simulink model "PassengerCar"  (R2019b)
settings: Solver=ode1  StartTime=0  StopTime=25  FixedStep=1.0000000000000000e-003  RelTol=1e-3
InitFcn:
  | sampleTime = str2double(get_param(bdroot, 'FixedStep'));
undefined symbols (not defined in the file or in its folder): AccPedalPos, BrakePedalPos, BrakeSwitch, DiscIntNeverNeededParam, DYNA4, EngSpd, IgnitionSwitch, InitialGear, InitialSpeed, IntendedEngTrq, LeftIndicator, MainBrakePress, MaxGear, MDL, MinGear, RefAcc, RefLane, RefLatPos, RefPath, RefPathCurv, RefSpd, RefSpdPreview, RefSpdRetrospect, RightIndicator, SteeringWheelAng, SteeringWheelTrq, UserDefinedRefValue, vm_const
libraries: UtilitiesLibrary x31, simulink x18, WheelSystemModules x13, LongitudinalControllerModules x13, LateralControllerModules x7, AnimationBusselectorModules x5, EnvironmentModules x5, BasicEngineControlModules x5, MiscellaneousControlModules x5, Animation3Modules x4, AuxiliariesModules x4, TireModules x4
(part 9 of 39)

== system PassengerCar/Vehicle/BrakeSystem/BrakeSystemPhysics ==
  fromBrakeControlCoordinator : Inport
  fromCTRL : Inport  Port=2
  fromBrakeSystemControlUnit : Inport  Port=3
  BrakeSystemPhysicsOutput : Subsystem  Tag=TESIS DYNAware Interface Block  mask{NeedsUpdate=off, SignalInfo=|}
      mask SignalInfo=|
      | {
      |   "Version": "4.6",
      |   "MuxedOutputBusName": "BrakeSystemPhysics",
      |   "MuxedInputBusName": "input",
      |   "MuxedInputSelected": false,
      |   "MuxedOutputSelected": true,
      |   "SignalData": [
      |     {
      |       "initialValue": "0.0",
      |       "name": "WheelBrakePressActive[0;1]",
      |       "comment": "",
      |       "minString": "",
      |       "maxString": "",
      |       "width": 1,
      |       "dataType": 0,
      |       "signalType": 0,
      |       "createSignal": false,
      |       "outputName": "WheelBrakePressActive[0;1]",
      |       "generateSignalAccessBlock": false,
      |       "accessId": "$(parentId).$(blockName).$(outputName)"
      |     },
      |     {
      |       "initialValue": "0.0",
      |       "name": "MaxMainBrakePress[Pa]",
      |       "comment": "",
      |       "minString": "",
      |       "maxString": "",
      |       "width": 1,
      |       "dataType": 0,
      |       "signalType": 0,
      |       "createSignal": false,
      |       "outputName": "MaxMainBrakePress[Pa]",
      |       "generateSignalAccessBlock": false,
      |       "accessId": "$(parentId).$(blockName).$(outputName)"
      |     },
      |     {
      |       "initialValue": "0.0",
      |       "name": "MainBrakePress[Pa]",
      |       "comment": "",
      |       "minString": "",
      |       "maxString": "",
      |       "width": 1,
      |       "dataType": 0,
      |       "signalType": 0,
      |       "createSignal": false,
      |       "outputName": "MainBrakePress[Pa]",
      |       "generateSignalAccessBlock": false,
      |       "accessId": "$(parentId).$(blockName).$(outputName)"
      |     },
      |     {
      |       "initialValue": "",
      |       "name": "FrontLeftWheelBrakePress[Pa]",
      |       "comment": "",
      |       "minString": "",
      |       "maxString": "",
      |       "width": 1,
      |       "dataType": 0,
      |       "signalType": 0,
      |       "createSignal": false,
      |       "outputName": "FrontLeftWheelBrakePress[Pa]",
      |       "generateSignalAccessBlock": false,
      |       "accessId": "$(parentId).$(blockName).$(outputName)"
      |     },
      |     {
      |       "initialValue": "",
      |       "name": "FrontRightWheelBrakePress[Pa]",
      |       "comment": "",
      |       "minString": "",
      |       "maxString": "",
      |       "width": 1,
      |       "dataType": 0,
      |       "signalType": 0,
      |       "createSignal": false,
      |       "outputName": "FrontRightWheelBrakePress[Pa]",
      |       "generateSignalAccessBlock": false,
      |       "accessId": "$(parentId).$(blockName).$(outputName)"
      |     },
      |     {
      |       "initialValue": "",
      |       "name": "RearLeftWheelBrakePress[Pa]",
      |       "comment": "",
      |       "minString": "",
      |       "maxString": "",
      |       "width": 1,
      |       "dataType": 0,
      |       "signalType": 0,
      |       "createSignal": false,
      |       "outputName": "RearLeftWheelBrakePress[Pa]",
      |       "generateSignalAccessBlock": false,
      |       "accessId": "$(parentId).$(blockName).$(outputName)"
      |     },
      |     {
      |       "initialValue": "",
      |       "name": "RearRightWheelBrakePress[Pa]",
      |       "comment": "",
      |       "minString": "",
      |       "maxString": "",
      |       "width": 1,
      |       "dataType": 0,
      |       "signalType": 0,
      |       "createSignal": false,
      |       "outputName": "RearRightWheelBrakePress[Pa]",
      |       "generateSignalAccessBlock": false,
      |       "accessId": "$(parentId).$(blockName).$(outputName)"
      |     },
      |     {
      |       "initialValue": "",
      |       "name": "Rear2LeftWheelBrakePress[Pa]",
      |       "comment": "",
      |       "minString": "",
      |       "maxString": "",
      |       "width": 1,
      |       "dataType": 0,
      |       "signalType": 0,
      |       "createSignal": false,
      |       "outputName": "Rear2LeftWheelBrakePress[Pa]",
      |       "generateSignalAccessBlock": false,
      |       "accessId": "$(parentId).$(blockName).$(outputName)"
      |     },
      |     {
      |       "initialValue": "",
      |       "name": "Rear2RightWheelBrakePress[Pa]",
      |       "comment": "",
      |       "minString": "",
      |       "maxString": "",
      |       "width": 1,
      |       "dataType": 0,
      |       "signalType": 0,
      |       "createSignal": false,
      |       "outputName": "Rear2RightWheelBrakePress[Pa]",
      |       "generateSignalAccessBlock": false,
      |       "accessId": "$(parentId).$(blockName).$(outputName)"
      |     },
      |     {
      |       "initialValue": "",
      |       "name": "Rear3LeftWheelBrakePress[Pa]",
      |       "comment": "",
      |       "minString": "",
      |       "maxString": "",
      |       "width": 1,
      |       "dataType": 0,
      |       "signalType": 0,
      |       "createSignal": false,
      |       "outputName": "Rear3LeftWheelBrakePress[Pa]",
      |       "generateSignalAccessBlock": false,
      |       "accessId": "$(parentId).$(blockName).$(outputName)"
      |     },
      |     {
      |       "initialValue": "",
      |       "name": "Rear3RightWheelBrakePress[Pa]",
      |       "comment": "",
      |       "minString": "",
      |       "maxString": "",
      |       "width": 1,
      |       "dataType": 0,
      |       "signalType": 0,
      |       "createSignal": false,
      |       "outputName": "Rear3RightWheelBrakePress[Pa]",
      |       "generateSignalAccessBlock": false,
      |       "accessId": "$(parentId).$(blockName).$(outputName)"
      |     }
      |   ]
      | }
      mask prompts: NeedsUpdate "Specify, if subsystem content needs to be updated"; SignalInfo "Signal Info (json)"
      mask help: DYNA4 Interface Block Version 4.6
      mask init:
      | blockName = get_param(gcbh, 'Name');
      | parentId = DYNA4.ModelHandling.AccessID.getFromHierarchy(gcbh);
      | TD.InterfaceBlock.ModelCallbacks.GenerateContent(gcb);
      settings: DeleteFcn=TD.InterfaceBlock.ModelCallbacks.CloseGUI( gcbh );  NameChangeFcn=TD.InterfaceBlock.ModelCallbacks.BlockRenamedHandler(gcbh);  OpenFcn=TD.InterfaceBlock.ModelCallbacks.OpenGUI( gcbh );  CloseFcn=TD.InterfaceBlock.ModelCallbacks.CloseGUI( gcbh );
      mask Display:
      | image('InterfaceBlock.png','center');
      | port_label('input',1, 'WheelBrakePressActive[0;1]');
      | port_label('input',2, 'MaxMainBrakePress[Pa]');
      | port_label('input',3, 'MainBrakePress[Pa]');
      | port_label('input',4, 'FrontLeftWheelBrakePress[Pa]');
      | port_label('input',5, 'FrontRightWheelBrakePress[Pa]');
      | port_label('input',6, 'RearLeftWheelBrakePress[Pa]');
      | port_label('input',7, 'RearRightWheelBrakePress[Pa]');
      | port_label('input',8, 'Rear2LeftWheelBrakePress[Pa]');
      | port_label('input',9, 'Rear2RightWheelBrakePress[Pa]');
      | port_label('input',10, 'Rear3LeftWheelBrakePress[Pa]');
      | port_label('input',11, 'Rear3RightWheelBrakePress[Pa]');
      | port_label('output',1, 'BrakeSystemPhysics');
  Compare To Constant : simulink/Logic and Bit Operations/Compare To Constant  relop=~=  const=double(DYNA4.Vehicle.BrakeSystem.BrakeSwitch.WHEEL_BRAKE_PRESSURES)  OutDataTypeStr=boolean
  Data Type Conversion : DataTypeConversion  OutDataTypeStr=double
  Demux : Demux  Outputs=8
  DynaComponentInfo : Subsystem  Tag=DynaComponentInfo
      mask init:
      | data= get_param(gcb, 'UserData');
      settings: OpenFcn=DYNA4.ModelHandling.Component.ShowEditComponentInformationDialog(gcb);
      mask Display: disp(['Type = ', data.type, '\nGroup = ', data.group, '\nName = ', data.name ])
  InputFromBrakeControlCoordinator : Subsystem  Tag=TESIS DYNAware Interface Block  mask{NeedsUpdate=off, SignalInfo=|}
      mask SignalInfo=|
      | {
      |   "Version": "4.6",
      |   "MuxedOutputBusName": "output",
      |   "MuxedInputBusName": "fromBrakeControlCoordinator",
      |   "MuxedInputSelected": true,
      |   "MuxedOutputSelected": false,
      |   "SignalData": [
      |     {
      |       "initialValue": "",
      |       "name": "BrakeSwitch[1;3]",
      |       "comment": "",
      |       "minString": "",
      |       "maxString": "",
      |       "width": -1,
      |       "dataType": 0,
      |       "signalType": 0,
      |       "createSignal": false,
      |       "outputName": "BrakeSwitch[1;3]",
      |       "generateSignalAccessBlock": false,
      |       "accessId": "$(parentId).$(blockName).$(outputName)"
      |     },
      |     {
      |       "initialValue": "",
      |       "name": "MainBrakePress[Pa]",
      |       "comment": "",
      |       "minString": "",
      |       "maxString": "",
      |       "width": -1,
      |       "dataType": 0,
      |       "signalType": 0,
      |       "createSignal": false,
      |       "outputName": "MainBrakePress[Pa]",
      |       "generateSignalAccessBlock": false,
      |       "accessId": "$(parentId).$(blockName).$(outputName)"
      |     }
      |   ]
      | }
      mask prompts: NeedsUpdate "Specify, if subsystem content needs to be updated"; SignalInfo "Signal Info (json)"
      mask help: DYNA4 Interface Block Version 4.6
      mask init:
      | blockName = get_param(gcbh, 'Name');
      | parentId = DYNA4.ModelHandling.AccessID.getFromHierarchy(gcbh);
      | TD.InterfaceBlock.ModelCallbacks.GenerateContent(gcb);
      settings: DeleteFcn=TD.InterfaceBlock.ModelCallbacks.CloseGUI( gcbh );  NameChangeFcn=TD.InterfaceBlock.ModelCallbacks.BlockRenamedHandler(gcbh);  OpenFcn=TD.InterfaceBlock.ModelCallbacks.OpenGUI( gcbh );  CloseFcn=TD.InterfaceBlock.ModelCallbacks.CloseGUI( gcbh );
      mask Display:
      | image('InterfaceBlock.png','center');
      | port_label('input',1, 'fromBrakeControlCoordinator');
      | port_label('output',1, 'BrakeSwitch[1;3]');
      | port_label('output',2, 'MainBrakePress[Pa]');
  InputFromCTRL : Subsystem  Tag=TESIS DYNAware Interface Block  mask{NeedsUpdate=off, SignalInfo=|}
      mask SignalInfo=|
      | {
      |   "Version": "4.6",
      |   "MuxedOutputBusName": "output",
      |   "MuxedInputBusName": "fromCTRL",
      |   "MuxedInputSelected": true,
      |   "MuxedOutputSelected": false,
      |   "SignalData": {
      |     "initialValue": "0.0",
      |     "name": "CTRL.LongitudinalControl.BrakePedalPos[0_1]",
      |     "comment": "",
      |     "minString": "",
      |     "maxString": "",
      |     "width": 1,
      |     "dataType": 0,
      |     "signalType": 0,
      |     "createSignal": false,
      |     "outputName": "BrakePedalPos[0_1]",
      |     "generateSignalAccessBlock": false,
      |     "accessId": "$(parentId).$(blockName).$(outputName)"
      |   }
      | }
      mask prompts: NeedsUpdate "Specify, if subsystem content needs to be updated"; SignalInfo "Signal Info (json)"
      mask help: DYNA4 Interface Block Version 4.6
      mask init:
      | blockName = get_param(gcbh, 'Name');
      | parentId = DYNA4.ModelHandling.AccessID.getFromHierarchy(gcbh);
      | TD.InterfaceBlock.ModelCallbacks.GenerateContent(gcb);
      settings: DeleteFcn=TD.InterfaceBlock.ModelCallbacks.CloseGUI( gcbh );  NameChangeFcn=TD.InterfaceBlock.ModelCallbacks.BlockRenamedHandler(gcbh);  OpenFcn=TD.InterfaceBlock.ModelCallbacks.OpenGUI( gcbh );  CloseFcn=TD.InterfaceBlock.ModelCallbacks.CloseGUI( gcbh );
      mask Display:
      | image('InterfaceBlock.png','center');
      | port_label('input',1, 'fromCTRL');
      | port_label('output',1, 'BrakePedalPos[0_1]');
  TabledBrakeHydraulics : BrakeSystemModules/TabledBrakeHydraulics  Tag=vedynaBrkHydMask  local_comp_inst=1  system_comp_inst=1  DATA_NODE=MDL.Vehicle.BrakeSystem.BrakeSystemPhysics.TabledBrakeHydraulics  sample_time=-1
  Terminator : Terminator
  BrakeSystemPhysics : Outport  VectorParamsAs1DForOutWhenUnconnected=off
  wires:
  Demux/1 -> BrakeSystemPhysicsOutput/4(FrontLeftWheelBrakePress[Pa]___UNIQUE_1)
  Demux/2 -> BrakeSystemPhysicsOutput/5(FrontRightWheelBrakePress[Pa]___UNIQUE_1)
  Demux/3 -> BrakeSystemPhysicsOutput/6(RearLeftWheelBrakePress[Pa]___UNIQUE_1)
  Demux/4 -> BrakeSystemPhysicsOutput/7(RearRightWheelBrakePress[Pa]___UNIQUE_1)
  Demux/5 -> BrakeSystemPhysicsOutput/8(Rear2LeftWheelBrakePress[Pa]___UNIQUE_1)
  Demux/6 -> BrakeSystemPhysicsOutput/9(Rear2RightWheelBrakePress[Pa]___UNIQUE_1)
  Demux/7 -> BrakeSystemPhysicsOutput/10(Rear3LeftWheelBrakePress[Pa]___UNIQUE_1)
  Demux/8 -> BrakeSystemPhysicsOutput/11(Rear3RightWheelBrakePress[Pa]___UNIQUE_1)
  InputFromCTRL/1(BrakePedalPos[0_1]___UNIQUE_1) -> TabledBrakeHydraulics/2
  fromCTRL/1 -> InputFromCTRL/1(fromCTRL)
  TabledBrakeHydraulics/3 -> Demux/1
  TabledBrakeHydraulics/2 -> BrakeSystemPhysicsOutput/3(MainBrakePress[Pa]___UNIQUE_1)
  TabledBrakeHydraulics/1 -> BrakeSystemPhysicsOutput/2(MaxMainBrakePress[Pa]___UNIQUE_1)
  BrakeSystemPhysicsOutput/1(BrakeSystemPhysics___UNIQUE_1) -> BrakeSystemPhysics/1
  fromBrakeControlCoordinator/1 -> InputFromBrakeControlCoordinator/1(fromBrakeControlCoordinator)
  InputFromBrakeControlCoordinator/1(BrakeSwitch[1;3]___UNIQUE_1) -> TabledBrakeHydraulics/1, Compare To Constant/1
  InputFromBrakeControlCoordinator/2(MainBrakePress[Pa]___UNIQUE_1) -> TabledBrakeHydraulics/3
  fromBrakeSystemControlUnit/1 -> Terminator/1
  Compare To Constant/1 -> Data Type Conversion/1
  Data Type Conversion/1 -> BrakeSystemPhysicsOutput/1(WheelBrakePressActive[0;1]___UNIQUE_1)

== system PassengerCar/Vehicle/BrakeSystem/BrakeSystemPhysicsOutput ==
  MaxMainBrakePress[Pa]___UNIQUE_1 : Inport  Description=|  PortDimensions=[1]
      | <name>MaxMainBrakePress[Pa]</name>
      | <comment></comment>
  MainBrakePress[Pa]___UNIQUE_1 : Inport  Description=|  Port=2  PortDimensions=[1]
      | <name>MainBrakePress[Pa]</name>
      | <comment></comment>
  FrontLeftWheelBrakePress[Pa]___UNIQUE_1 : Inport  Description=|  Port=3
      | <name>FrontLeftWheelBrakePress[Pa]</name>
      | <comment></comment>
  FrontRightWheelBrakePress[Pa]___UNIQUE_1 : Inport  Description=|  Port=4
      | <name>FrontRightWheelBrakePress[Pa]</name>
      | <comment></comment>
  RearLeftWheelBrakePress[Pa]___UNIQUE_1 : Inport  Description=|  Port=5
      | <name>RearLeftWheelBrakePress[Pa]</name>
      | <comment></comment>
  RearRightWheelBrakePress[Pa]___UNIQUE_1 : Inport  Description=|  Port=6
      | <name>RearRightWheelBrakePress[Pa]</name>
      | <comment></comment>
  Rear2LeftWheelBrakePress[Pa]___UNIQUE_1 : Inport  Description=|  Port=7
      | <name>Rear2LeftWheelBrakePress[Pa]</name>
      | <comment></comment>
  Rear2RightWheelBrakePress[Pa]___UNIQUE_1 : Inport  Description=|  Port=8
      | <name>Rear2RightWheelBrakePress[Pa]</name>
      | <comment></comment>
  Rear3LeftWheelBrakePress[Pa]___UNIQUE_1 : Inport  Description=|  Port=9
      | <name>Rear3LeftWheelBrakePress[Pa]</name>
      | <comment></comment>
  Rear3RightWheelBrakePress[Pa]___UNIQUE_1 : Inport  Description=|  Port=10
      | <name>Rear3RightWheelBrakePress[Pa]</name>
      | <comment></comment>
  WheelBrakePressSource[-]___UNIQUE_1 : Inport  Description=|  Port=11  PortDimensions=[1]
      | <name>WheelBrakePressSource[-]</name>
      | <comment></comment>
  __TDD__BrakeSystem.FrontLeftWheelBrakePress[Pa] : Demux  Outputs=1
  __TDD__BrakeSystem.FrontRightWheelBrakePress[Pa] : Demux  Outputs=1
  __TDD__BrakeSystem.MainBrakePress[Pa] : Demux  Outputs=[1]
  __TDD__BrakeSystem.MaxMainBrakePress[Pa] : Demux  Outputs=[1]
  __TDD__BrakeSystem.Rear2LeftWheelBrakePress[Pa] : Demux  Outputs=1
  __TDD__BrakeSystem.Rear2RightWheelBrakePress[Pa] : Demux  Outputs=1
  __TDD__BrakeSystem.Rear3LeftWheelBrakePress[Pa] : Demux  Outputs=1
  __TDD__BrakeSystem.Rear3RightWheelBrakePress[Pa] : Demux  Outputs=1
  __TDD__BrakeSystem.RearLeftWheelBrakePress[Pa] : Demux  Outputs=1
  __TDD__BrakeSystem.RearRightWheelBrakePress[Pa] : Demux  Outputs=1
  __TDD__BrakeSystem.WheelBrakePressSource[-] : Demux  Outputs=[1]
  __TDO__BrakeSystem : BusCreator  Inputs=11
  BrakeSystem___UNIQUE_1 : Outport  Description=|  VectorParamsAs1DForOutWhenUnconnected=off
      | <name>MaxMainBrakePress[Pa]</name>
      | <comment></comment>
  wires:
  MaxMainBrakePress[Pa]___UNIQUE_1/1 -> __TDD__BrakeSystem.MaxMainBrakePress[Pa]/1  "MaxMainBrakePress[Pa]"
  __TDD__BrakeSystem.MaxMainBrakePress[Pa]/1 -> __TDO__BrakeSystem/1  "MaxMainBrakePress[Pa]"
  MainBrakePress[Pa]___UNIQUE_1/1 -> __TDD__BrakeSystem.MainBrakePress[Pa]/1  "MainBrakePress[Pa]"
  __TDD__BrakeSystem.MainBrakePress[Pa]/1 -> __TDO__BrakeSystem/2  "MainBrakePress[Pa]"
  FrontLeftWheelBrakePress[Pa]___UNIQUE_1/1 -> __TDD__BrakeSystem.FrontLeftWheelBrakePress[Pa]/1  "FrontLeftWheelBrakePress[Pa]"
  __TDD__BrakeSystem.FrontLeftWheelBrakePress[Pa]/1 -> __TDO__BrakeSystem/3  "FrontLeftWheelBrakePress[Pa]"
  FrontRightWheelBrakePress[Pa]___UNIQUE_1/1 -> __TDD__BrakeSystem.FrontRightWheelBrakePress[Pa]/1  "FrontRightWheelBrakePress[Pa]"
  __TDD__BrakeSystem.FrontRightWheelBrakePress[Pa]/1 -> __TDO__BrakeSystem/4  "FrontRightWheelBrakePress[Pa]"
  RearLeftWheelBrakePress[Pa]___UNIQUE_1/1 -> __TDD__BrakeSystem.RearLeftWheelBrakePress[Pa]/1  "RearLeftWheelBrakePress[Pa]"
  __TDD__BrakeSystem.RearLeftWheelBrakePress[Pa]/1 -> __TDO__BrakeSystem/5  "RearLeftWheelBrakePress[Pa]"
  RearRightWheelBrakePress[Pa]___UNIQUE_1/1 -> __TDD__BrakeSystem.RearRightWheelBrakePress[Pa]/1  "RearRightWheelBrakePress[Pa]"
  __TDD__BrakeSystem.RearRightWheelBrakePress[Pa]/1 -> __TDO__BrakeSystem/6  "RearRightWheelBrakePress[Pa]"
  Rear2LeftWheelBrakePress[Pa]___UNIQUE_1/1 -> __TDD__BrakeSystem.Rear2LeftWheelBrakePress[Pa]/1  "Rear2LeftWheelBrakePress[Pa]"
  __TDD__BrakeSystem.Rear2LeftWheelBrakePress[Pa]/1 -> __TDO__BrakeSystem/7  "Rear2LeftWheelBrakePress[Pa]"
  Rear2RightWheelBrakePress[Pa]___UNIQUE_1/1 -> __TDD__BrakeSystem.Rear2RightWheelBrakePress[Pa]/1  "Rear2RightWheelBrakePress[Pa]"
  __TDD__BrakeSystem.Rear2RightWheelBrakePress[Pa]/1 -> __TDO__BrakeSystem/8  "Rear2RightWheelBrakePress[Pa]"
  Rear3LeftWheelBrakePress[Pa]___UNIQUE_1/1 -> __TDD__BrakeSystem.Rear3LeftWheelBrakePress[Pa]/1  "Rear3LeftWheelBrakePress[Pa]"
  __TDD__BrakeSystem.Rear3LeftWheelBrakePress[Pa]/1 -> __TDO__BrakeSystem/9  "Rear3LeftWheelBrakePress[Pa]"
  Rear3RightWheelBrakePress[Pa]___UNIQUE_1/1 -> __TDD__BrakeSystem.Rear3RightWheelBrakePress[Pa]/1  "Rear3RightWheelBrakePress[Pa]"
  __TDD__BrakeSystem.Rear3RightWheelBrakePress[Pa]/1 -> __TDO__BrakeSystem/10  "Rear3RightWheelBrakePress[Pa]"
  WheelBrakePressSource[-]___UNIQUE_1/1 -> __TDD__BrakeSystem.WheelBrakePressSource[-]/1
  __TDD__BrakeSystem.WheelBrakePressSource[-]/1 -> __TDO__BrakeSystem/11  "WheelBrakePressSource[-]"
  __TDO__BrakeSystem/1 -> BrakeSystem___UNIQUE_1/1  "BrakeSystem"

== system PassengerCar/Vehicle/BrakeSystem/DynaComponentInfo ==

== system PassengerCar/Vehicle/BrakeSystem/Signal Prioritizer ==
  BrakeControlCoordinator : Inport
  BrakeSystemControlUnit : Inport  Port=2
  BrakeSystemPhysics : Inport  Port=3
  Add : Sum
  Bus Creator : BusCreator  Inputs=8
  Bus Selector : BusSelector  OutputSignals=FrontLeftWheelBrakePress[Pa],FrontRightWheelBrakePress[Pa],RearLeftWheelBrakePress[Pa],RearRightWheelBrakePress[Pa],Rear2LeftWheelBrakePress[Pa],Rear2RightWheelBrakePress[Pa],Rear3LeftWheelBrakePress[Pa],Rear3RightWheelBrakePress[Pa],WheelBrakePressActive[0;1]
  Bus Selector1 : BusSelector  OutputSignals=FrontLeftWheelBrakePress[Pa],FrontRightWheelBrakePress[Pa],RearLeftWheelBrakePress[Pa],RearRightWheelBrakePress[Pa],Rear2LeftWheelBrakePress[Pa],Rear2RightWheelBrakePress[Pa],Rear3LeftWheelBrakePress[Pa],Rear3RightWheelBrakePress[Pa],WheelBrakePressActive[0;1]
  Bus Selector2 : BusSelector  OutputSignals=FrontLeftWheelBrakePress[Pa],FrontRightWheelBrakePress[Pa],RearLeftWheelBrakePress[Pa],RearRightWheelBrakePress[Pa],Rear2LeftWheelBrakePress[Pa],Rear2RightWheelBrakePress[Pa],Rear3LeftWheelBrakePress[Pa],Rear3RightWheelBrakePress[Pa],WheelBrakePressActive[0;1]
  Compare To Zero : simulink/Logic and Bit Operations/Compare To Zero  relop===  OutDataTypeStr=boolean
  Constant : Constant  Value=1:4
  Constant1 : Constant  Value=[1:3, -1]
  Constant2 : Constant
  Constant3 : Constant  Value=zeros(8,1)  VectorParams1D=off
  Demux : Demux  Outputs=8
  Gain : Gain  Gain=4
  MinMax : MinMax
  Product : Product  Tag=productActive
  Selector : Selector  NumberOfDimensions=2  InputPortWidth=3  IndexOptions=Select all,Starting index (port)  Indices=[1 3]  OutputSizes=1,1
  Selector1 : Selector  NumberOfDimensions=2  InputPortWidth=3  IndexOptions=Select all,Starting index (port)  Indices=[1 3]  OutputSizes=1,1
  Vector Concatenate : Concatenate  NumInputs=4
  Vector Concatenate1 : Concatenate  NumInputs=4  Mode=Multidimensional array  ConcatenateDimension=2
  Vector Concatenate2 : Concatenate  NumInputs=8
  Vector Concatenate3 : Concatenate  NumInputs=8
  Vector Concatenate4 : Concatenate  NumInputs=8
  ControlSignals : Outport  VectorParamsAs1DForOutWhenUnconnected=off
  SelectedInput : Outport  Port=2  VectorParamsAs1DForOutWhenUnconnected=off
  wires:
  Vector Concatenate4/1 -> Vector Concatenate1/3
  Bus Selector2/9 -> Vector Concatenate/3  "<WheelBrakePressActive[0;1]>"
  BrakeSystemPhysics/1 -> Bus Selector2/1
  Bus Selector2/8 -> Vector Concatenate4/8  "<Rear3RightWheelBrakePress[Pa]>"
  Bus Selector2/7 -> Vector Concatenate4/7  "<Rear3LeftWheelBrakePress[Pa]>"
  Bus Selector2/6 -> Vector Concatenate4/6  "<Rear2RightWheelBrakePress[Pa]>"
  Bus Selector2/5 -> Vector Concatenate4/5  "<Rear2LeftWheelBrakePress[Pa]>"
  Bus Selector2/4 -> Vector Concatenate4/4  "<RearRightWheelBrakePress[Pa]>"
  Bus Selector2/3 -> Vector Concatenate4/3  "<RearLeftWheelBrakePress[Pa]>"
  Bus Selector2/2 -> Vector Concatenate4/2  "<FrontRightWheelBrakePress[Pa]>"
  Bus Selector2/1 -> Vector Concatenate4/1  "<FrontLeftWheelBrakePress[Pa]>"
  Vector Concatenate3/1 -> Vector Concatenate1/2
  Bus Selector1/9 -> Vector Concatenate/2  "<WheelBrakePressActive[0;1]>"
  BrakeSystemControlUnit/1 -> Bus Selector1/1
  Bus Selector1/8 -> Vector Concatenate3/8  "<Rear3RightWheelBrakePress[Pa]>"
  Bus Selector1/7 -> Vector Concatenate3/7  "<Rear3LeftWheelBrakePress[Pa]>"
  Bus Selector1/6 -> Vector Concatenate3/6  "<Rear2RightWheelBrakePress[Pa]>"
  Bus Selector1/5 -> Vector Concatenate3/5  "<Rear2LeftWheelBrakePress[Pa]>"
  Bus Selector1/4 -> Vector Concatenate3/4  "<RearRightWheelBrakePress[Pa]>"
  Bus Selector1/3 -> Vector Concatenate3/3  "<RearLeftWheelBrakePress[Pa]>"
  Bus Selector1/2 -> Vector Concatenate3/2  "<FrontRightWheelBrakePress[Pa]>"
  Bus Selector1/1 -> Vector Concatenate3/1  "<FrontLeftWheelBrakePress[Pa]>"
  Vector Concatenate2/1 -> Vector Concatenate1/1
  Bus Selector/9 -> Vector Concatenate/1  "<WheelBrakePressActive[0;1]>"
  BrakeControlCoordinator/1 -> Bus Selector/1
  Bus Selector/8 -> Vector Concatenate2/8  "<Rear3RightWheelBrakePress[Pa]>"
  Bus Selector/7 -> Vector Concatenate2/7  "<Rear3LeftWheelBrakePress[Pa]>"
  Bus Selector/6 -> Vector Concatenate2/6  "<Rear2RightWheelBrakePress[Pa]>"
  Bus Selector/5 -> Vector Concatenate2/5  "<Rear2LeftWheelBrakePress[Pa]>"
  Bus Selector/4 -> Vector Concatenate2/4  "<RearRightWheelBrakePress[Pa]>"
  Bus Selector/3 -> Vector Concatenate2/3  "<RearLeftWheelBrakePress[Pa]>"
  Bus Selector/2 -> Vector Concatenate2/2  "<FrontRightWheelBrakePress[Pa]>"
  Bus Selector/1 -> Vector Concatenate2/1  "<FrontLeftWheelBrakePress[Pa]>"
  Vector Concatenate1/1 -> Selector/1
  Vector Concatenate/1 -> Product/2
  Constant2/1 -> Vector Concatenate/4
  Constant3/1 -> Vector Concatenate1/4
  Demux/8 -> Bus Creator/8  "Rear3RightWheelBrakePress[Pa]"
  Demux/7 -> Bus Creator/7  "Rear3LeftWheelBrakePress[Pa]"
  Demux/6 -> Bus Creator/6  "Rear2RightWheelBrakePress[Pa]"
  Demux/5 -> Bus Creator/5  "Rear2LeftWheelBrakePress[Pa]"
  Demux/4 -> Bus Creator/4  "RearRightWheelBrakePress[Pa]"
  Demux/3 -> Bus Creator/3  "RearLeftWheelBrakePress[Pa]"
  Demux/2 -> Bus Creator/2  "FrontRightWheelBrakePress[Pa]"
  Demux/1 -> Bus Creator/1  "FrontLeftWheelBrakePress[Pa]"
  Selector1/1 -> SelectedInput/1
  Bus Creator/1 -> ControlSignals/1
  Selector/1 -> Demux/1
  MinMax/1 -> Selector/2, Selector1/2
  Add/1 -> MinMax/1
  Gain/1 -> Add/1
  Compare To Zero/1 -> Gain/1
  Product/1 -> Compare To Zero/1, Add/2
  Constant/1 -> Product/1
  Constant1/1 -> Selector1/1

== system PassengerCar/Vehicle/Chassis/ComponentSpecificChassisInputs ==
  Ground : Ground
  Ground1 : Ground
  SteeringInputs : Outport  VectorParamsAs1DForOutWhenUnconnected=off
  ActuatedTrackRodInputs : Outport  Port=2  VectorParamsAs1DForOutWhenUnconnected=off
  wires:
  Ground1/1 -> ActuatedTrackRodInputs/1
  Ground/1 -> SteeringInputs/1

== system PassengerCar/Vehicle/Chassis/DynaComponentInfo ==

== system PassengerCar/Vehicle/CoolingSystem/CoolingSystemOutput ==
  NoCoolingSystem___UNIQUE_1 : Inport  Description=|  PortDimensions=[1]
      | <name>NoCoolingSystem</name>
      | <comment></comment>
  __TDD__CoolingSystem.NoCoolingSystem : Demux  Outputs=[1]
  __TDO__CoolingSystem : BusCreator  Inputs=1
  CoolingSystem___UNIQUE_1 : Outport  Description=|  PortDimensions=[1]  VectorParamsAs1DForOutWhenUnconnected=off
      | <name>NoCoolingSystem</name>
      | <comment></comment>
  wires:
  __TDO__CoolingSystem/1 -> CoolingSystem___UNIQUE_1/1  "CoolingSystem"
  __TDD__CoolingSystem.NoCoolingSystem/1 -> __TDO__CoolingSystem/1  "NoCoolingSystem"
  NoCoolingSystem___UNIQUE_1/1 -> __TDD__CoolingSystem.NoCoolingSystem/1

== system PassengerCar/Vehicle/CoolingSystem/DynaComponentInfo ==

== system PassengerCar/Vehicle/Drivetrain/DrivetrainControlUnit ==
  fromDrivetrainPhysics : Inport
  fromCTRL : Inport  Port=2
  fromEngine : Inport  Port=3
  DrivetrainControlUnitOutput : Subsystem  Tag=TESIS DYNAware Interface Block  mask{NeedsUpdate=off, SignalInfo=|}
      mask SignalInfo=|
      | {
      |   "Version": "4.6",
      |   "MuxedOutputBusName": "DrivetrainControlUnit",
      |   "MuxedInputBusName": "input",
      |   "MuxedInputSelected": false,
      |   "MuxedOutputSelected": true,
      |   "SignalData": [
      |     {
      |       "initialValue": "0.0",
      |       "name": "TransmissionControlUnit.Gear[-4;20]",
      |       "comment": "Gear",
      |       "minString": "",
      |       "maxString": "",
      |       "width": 1,
      |       "dataType": 0,
      |       "signalType": 0,
      |       "createSignal": false,
      |       "outputName": "TransmissionControlUnit.Gear[-4;20]",
      |       "generateSignalAccessBlock": false,
      |       "accessId": "$(parentId).$(blockName).$(outputName)"
      |     },
      |     {
      |       "initialValue": "0.0",
      |       "name": "TransmissionControlUnit.LockUpClutchPos[0_1]",
      |       "comment": "Lock-up clutch position",
      |       "minString": "",
      |       "maxString": "",
      |       "width": 1,
      |       "dataType": 0,
      |       "signalType": 0,
      |       "createSignal": false,
      |       "outputName": "TransmissionControlUnit.LockUpClutchPos[0_1]",
      |       "generateSignalAccessBlock": false,
      |       "accessId": "$(parentId).$(blockName).$(outputName)"
      |     },
      |     {
      |       "initialValue": "0.0",
      |       "name": "TransmissionControlUnit.AutomatedManualClutchPos[0_1]",
      |       "comment": "Clutch position for manual shifting",
      |       "minString": "",
      |       "maxString": "",
      |       "width": 1,
      |       "dataType": 0,
      |       "signalType": 0,
      |       "createSignal": false,
      |       "outputName": "TransmissionControlUnit.AutomatedManualClutchPos[0_1]",
      |       "generateSignalAccessBlock": false,
      |       "accessId": "$(parentId).$(blockName).$(outputName)"
      |     },
      |     {
      |       "initialValue": "0.0",
      |       "name": "TransmissionControlUnit.GearTarget[-4;20]",
      |       "comment": "Target gear",
      |       "minString": "",
      |       "maxString": "",
      |       "width": 1,
      |       "dataType": 0,
      |       "signalType": 0,
      |       "createSignal": false,
      |       "outputName": "TransmissionControlUnit.GearTarget[-4;20]",
      |       "generateSignalAccessBlock": false,
      |       "accessId": "$(parentId).$(blockName).$(outputName)"
      |     },
      |     {
      |       "initialValue": "0.0",
      |       "name": "TransmissionControlUnit.ASRRequestSwitch[0;2]",
      |       "comment": "",
      |       "minString": "",
      |       "maxString": "",
      |       "width": 1,
      |       "dataType": 0,
      |       "signalType": 0,
      |       "createSignal": false,
      |       "outputName": "TransmissionControlUnit.ASRRequestSwitch[0;2]",
      |       "generateSignalAccessBlock": false,
      |       "accessId": "$(parentId).$(blockName).$(outputName)"
      |     },
      |     {
      |       "initialValue": "0.0",
      |       "name": "TransmissionControlUnit.ASRTrq[Nm]",
      |       "comment": "",
      |       "minString": "",
      |       "maxString": "",
      |       "width": 1,
      |       "dataType": 0,
      |       "signalType": 0,
      |       "createSignal": false,
      |       "outputName": "TransmissionControlUnit.ASRTrq[Nm]",
      |       "generateSignalAccessBlock": false,
      |       "accessId": "$(parentId).$(blockName).$(outputName)"
      |     },
      |     {
      |       "initialValue": "0.0",
      |       "name": "",
      |       "comment": "",
      |       "minString": "",
      |       "maxString": "",
      |       "width": 1,
      |       "dataType": 0,
      |       "signalType": 0,
      |       "createSignal": true,
      |       "outputName": "TransmissionControlUnit.MSRRequestSwitch[0;2]",
      |       "generateSignalAccessBlock": false,
      |       "accessId": "$(parentId).$(blockName).$(outputName)"
      |     },
      |     {
      |       "initialValue": "0.0",
      |       "name": "",
      |       "comment": "",
      |       "minString": "",
      |       "maxString": "",
      |       "width": 1,
      |       "dataType": 0,
      |       "signalType": 0,
      |       "createSignal": true,
      |       "outputName": "TransmissionControlUnit.MSRTrq[Nm]",
      |       "generateSignalAccessBlock": false,
      |       "accessId": "$(parentId).$(blockName).$(outputName)"
      |     }
      |   ]
      | }
      mask prompts: NeedsUpdate "Specify, if subsystem content needs to be updated"; SignalInfo "Signal Info (json)"
      mask help: DYNA4 Interface Block Version 4.6
      mask init:
      | blockName = get_param(gcbh, 'Name');
      | parentId = DYNA4.ModelHandling.AccessID.getFromHierarchy(gcbh);
      | TD.InterfaceBlock.ModelCallbacks.GenerateContent(gcb);
      settings: DeleteFcn=TD.InterfaceBlock.ModelCallbacks.CloseGUI( gcbh );  NameChangeFcn=TD.InterfaceBlock.ModelCallbacks.BlockRenamedHandler(gcbh);  OpenFcn=TD.InterfaceBlock.ModelCallbacks.OpenGUI( gcbh );  CloseFcn=TD.InterfaceBlock.ModelCallbacks.CloseGUI( gcbh );
      settings: AttributesFormatString=|
      | TransmissionControlUnit.MSRRequestSwitch[0;2] = 0.0
      | TransmissionControlUnit.MSRTrq[Nm] = 0.0
      mask Display:
      | image('InterfaceBlock.png','center');
      | port_label('input',1, 'TransmissionControlUnit.Gear[-4;20]');
      | port_label('input',2, 'TransmissionControlUnit.LockUpClutchPos[0_1]');
      | port_label('input',3, 'TransmissionControlUnit.AutomatedManualClutchPos[0_1]');
      | port_label('input',4, 'TransmissionControlUnit.GearTarget[-4;20]');
      | port_label('input',5, 'TransmissionControlUnit.ASRRequestSwitch[0;2]');
      | port_label('input',6, 'TransmissionControlUnit.ASRTrq[Nm]');
      | port_label('output',1, 'DrivetrainControlUnit');
  DynaComponentInfo : Subsystem  Tag=DynaComponentInfo
      mask init:
      | data= get_param(gcb, 'UserData');
      settings: OpenFcn=DYNA4.ModelHandling.Component.ShowEditComponentInformationDialog(gcb);
      mask Display: disp(['Type = ', data.type, '\nGroup = ', data.group, '\nName = ', data.name ])
  InputFromCTRL : Subsystem  Tag=TESIS DYNAware Interface Block  mask{NeedsUpdate=off, SignalInfo=|}
      mask SignalInfo=|
      | {
      |   "Version": "4.6",
      |   "MuxedOutputBusName": "Drivetrain",
      |   "MuxedInputBusName": "fromCTRL",
      |   "MuxedInputSelected": true,
      |   "MuxedOutputSelected": false,
      |   "SignalData": [
      |     {
      |       "initialValue": "0.0",
      |       "name": "CTRL.LongitudinalControl.TransmissionLoad[0_1]",
      |       "comment": "",
      |       "minString": "",
      |       "maxString": "",
      |       "width": 1,
      |       "dataType": 0,
      |       "signalType": 0,
      |       "createSignal": false,
      |       "outputName": "TransmissionLoad[0_1]",
      |       "generateSignalAccessBlock": false,
      |       "accessId": "$(parentId).$(blockName).$(outputName)"
      |     },
      |     {
      |       "initialValue": "0.0",
      |       "name": "CTRL.LongitudinalControl.IntendedEngTrqActive[0;1]",
      |       "comment": "",
      |       "minString": "",
      |       "maxString": "",
      |       "width": 1,
      |       "dataType": 0,
      |       "signalType": 0,
      |       "createSignal": false,
      |       "outputName": "IntendedEngTrqActive[0;1]",
      |       "generateSignalAccessBlock": false,
      |       "accessId": "$(parentId).$(blockName).$(outputName)"
      |     },
      |     {
      |       "initialValue": "0.0",
      |       "name": "CTRL.LongitudinalControl.AccPedalPos[0_1]",
      |       "comment": "",
      |       "minString": "",
      |       "maxString": "",
      |       "width": 1,
      |       "dataType": 0,
      |       "signalType": 0,
      |       "createSignal": false,
      |       "outputName": "AccPedalPos[0_1]",
      |       "generateSignalAccessBlock": false,
      |       "accessId": "$(parentId).$(blockName).$(outputName)"
      |     },
      |     {
      |       "initialValue": "0.0",
      |       "name": "CTRL.LongitudinalControl.InitialGear[-4;20]",
      |       "comment": "",
      |       "minString": "",
      |       "maxString": "",
      |       "width": 1,
      |       "dataType": 0,
      |       "signalType": 0,
      |       "createSignal": false,
      |       "outputName": "InitialGear[-4;20]",
      |       "generateSignalAccessBlock": false,
      |       "accessId": "$(parentId).$(blockName).$(outputName)"
      |     },
      |     {
      |       "initialValue": "0.0",
      |       "name": "CTRL.LongitudinalControl.MaxGear[-4;20]",
      |       "comment": "Maximum gear",
      |       "minString": "",
      |       "maxString": "",
      |       "width": 1,
      |       "dataType": 0,
      |       "signalType": 0,
      |       "createSignal": false,
      |       "outputName": "MaxGear[-4;20]",
      |       "generateSignalAccessBlock": false,
      |       "accessId": "$(parentId).$(blockName).$(outputName)"
      |     },
      |     {
      |       "initialValue": "0.0",
      |       "name": "CTRL.LongitudinalControl.MinGear[-4;20]",
      |       "comment": "Minimum gear",
      |       "minString": "",
      |       "maxString": "",
      |       "width": 1,
      |       "dataType": 0,
      |       "signalType": 0,
      |       "createSignal": false,
      |       "outputName": "MinGear[-4;20]",
      |       "generateSignalAccessBlock": false,
      |       "accessId": "$(parentId).$(blockName).$(outputName)"
      |     },
      |     {
      |       "initialValue": "0.0",
      |       "name": "CTRL.LongitudinalControl.ShiftingProgramSelection[-]",
      |       "comment": "Shifting program selection",
      |       "minString": "",
      |       "maxString": "",
      |       "width": 1,
      |       "dataType": 0,
      |       "signalType": 0,
      |       "createSignal": false,
      |       "outputName": "ShiftingProgramSelection[-]",
      |       "generateSignalAccessBlock": false,
      |       "accessId": "$(parentId).$(blockName).$(outputName)"
      |     },
      |     {
      |       "initialValue": "0.0",
      |       "name": "CTRL.LongitudinalControl.KickdownSwitch[0;1]",
      |       "comment": "Kickdown switch",
      |       "minString": "",
      |       "maxString": "",
      |       "width": 1,
      |       "dataType": 0,
      |       "signalType": 0,
      |       "createSignal": false,
      |       "outputName": "KickdownSwitch[0;1]",
      |       "generateSignalAccessBlock": false,
      |       "accessId": "$(parentId).$(blockName).$(outputName)"
      |     }
      |   ]
      | }
      mask prompts: NeedsUpdate "Specify, if subsystem content needs to be updated"; SignalInfo "Signal Info (json)"
      mask help: DYNA4 Interface Block Version 4.6
      mask init:
      | blockName = get_param(gcbh, 'Name');
      | parentId = DYNA4.ModelHandling.AccessID.getFromHierarchy(gcbh);
      | TD.InterfaceBlock.ModelCallbacks.GenerateContent(gcb);
      settings: DeleteFcn=TD.InterfaceBlock.ModelCallbacks.CloseGUI( gcbh );  NameChangeFcn=TD.InterfaceBlock.ModelCallbacks.BlockRenamedHandler(gcbh);  OpenFcn=TD.InterfaceBlock.ModelCallbacks.OpenGUI( gcbh );  CloseFcn=TD.InterfaceBlock.ModelCallbacks.CloseGUI( gcbh );
      mask Display:
      | image('InterfaceBlock.png','center');
      | port_label('input',1, 'fromCTRL');
      | port_label('output',1, 'TransmissionLoad[0_1]');
      | port_label('output',2, 'IntendedEngTrqActive[0;1]');
      | port_label('output',3, 'AccPedalPos[0_1]');
      | port_label('output',4, 'InitialGear[-4;20]');
      | port_label('output',5, 'MaxGear[-4;20]');
      | port_label('output',6, 'MinGear[-4;20]');
      | port_label('output',7, 'ShiftingProgramSelection[-]');
      | port_label('output',8, 'KickdownSwitch[0;1]');
  InputFromDrivetrainPhysics : Subsystem  Tag=TESIS DYNAware Interface Block  mask{NeedsUpdate=off, SignalInfo=|}
      mask SignalInfo=|
      | {
      |   "Version": "4.6",
      |   "MuxedOutputBusName": "Drivetrain",
      |   "MuxedInputBusName": "fromDrivetrainPhysics",
      |   "MuxedInputSelected": true,
      |   "MuxedOutputSelected": false,
      |   "SignalData": [
      |     {
      |       "initialValue": "0.0",
      |       "name": "Transmission.Type[-]",
      |       "comment": "",
      |       "minString": "",
      |       "maxString": "",
      |       "width": -1,
      |       "dataType": 0,
      |       "signalType": 0,
      |       "createSignal": false,
      |       "outputName": "Type[-]",
      |       "generateSignalAccessBlock": false,
      |       "accessId": "$(parentId).$(blockName).$(outputName)"
      |     },
      |     {
      |       "initialValue": "0.0",
      |       "name": "EngSpd[rad/s]",
      |       "comment": "Engine speed",
      |       "minString": "",
      |       "maxString": "",
      |       "width": 1,
      |       "dataType": 0,
      |       "signalType": 0,
      |       "createSignal": false,
      |       "outputName": "EngSpd[rad/s]",
      |       "generateSignalAccessBlock": false,
      |       "accessId": "$(parentId).$(blockName).$(outputName)"
      |     },
      |     {
      |       "initialValue": "0.0",
      |       "name": "Transmission.InSpd[rad/s]",
      |       "comment": "Transmission input speed",
      |       "minString": "",
      |       "maxString": "",
      |       "width": 1,
      |       "dataType": 0,
      |       "signalType": 0,
      |       "createSignal": false,
      |       "outputName": "InSpd[rad/s]",
      |       "generateSignalAccessBlock": false,
      |       "accessId": "$(parentId).$(blockName).$(outputName)"
      |     },
      |     {
      |       "initialValue": "0.0",
      |       "name": "Transmission.OutSpd[rad/s]",
      |       "comment": "Transmission output speed",
      |       "minString": "",
      |       "maxString": "",
      |       "width": 1,
      |       "dataType": 0,
      |       "signalType": 0,
      |       "createSignal": false,
      |       "outputName": "OutSpd[rad/s]",
      |       "generateSignalAccessBlock": false,
      |       "accessId": "$(parentId).$(blockName).$(outputName)"
      |     },
      |     {
      |       "initialValue": "0.0",
      |       "name": "Transmission.NumFwdGears[-]",
      |       "comment": "Number of forward gears",
      |       "minString": "",
      |       "maxString": "",
      |       "width": 1,
      |       "dataType": 0,
      |       "signalType": 0,
      |       "createSignal": false,
      |       "outputName": "NumFwdGears[-]",
      |       "generateSignalAccessBlock": false,
      |       "accessId": "$(parentId).$(blockName).$(outputName)"
      |     }
      |   ]
      | }
      mask prompts: NeedsUpdate "Specify, if subsystem content needs to be updated"; SignalInfo "Signal Info (json)"
      mask help: DYNA4 Interface Block Version 4.6
      mask init:
      | blockName = get_param(gcbh, 'Name');
      | parentId = DYNA4.ModelHandling.AccessID.getFromHierarchy(gcbh);
      | TD.InterfaceBlock.ModelCallbacks.GenerateContent(gcb);
      settings: DeleteFcn=TD.InterfaceBlock.ModelCallbacks.CloseGUI( gcbh );  NameChangeFcn=TD.InterfaceBlock.ModelCallbacks.BlockRenamedHandler(gcbh);  OpenFcn=TD.InterfaceBlock.ModelCallbacks.OpenGUI( gcbh );  CloseFcn=TD.InterfaceBlock.ModelCallbacks.CloseGUI( gcbh );
      mask Display:
      | image('InterfaceBlock.png','center');
      | port_label('input',1, 'fromDrivetrainPhysics');
      | port_label('output',1, 'Type[-]');
      | port_label('output',2, 'EngSpd[rad/s]');
      | port_label('output',3, 'InSpd[rad/s]');
      | port_label('output',4, 'OutSpd[rad/s]');
      | port_label('output',5, 'NumFwdGears[-]');
  Switch : Switch  Criteria=u2 > Threshold
  Terminator : Terminator
  Transmission.Type ~= Manual : simulink/Logic and Bit Operations/Compare To Constant  relop=>  const=double(DYNA4.Vehicle.Drivetrain.DrivetrainPhysics.TransmissionType.MANUAL)  OutDataTypeStr=boolean  ZeroCross=off
  TransmissionControlUnit : Subsystem
  DrivetrainControlUnit : Outport  VectorParamsAs1DForOutWhenUnconnected=off
  wires:
  DrivetrainControlUnitOutput/1(DrivetrainControlUnit___UNIQUE_1) -> DrivetrainControlUnit/1
  TransmissionControlUnit/3(AutomatedManualClutchPos[0_1]) -> DrivetrainControlUnitOutput/3(AutomatedManualClutchPos[0_1]___UNIQUE_1)
  TransmissionControlUnit/4(GearTarget[-4;20]) -> DrivetrainControlUnitOutput/4(GearTarget[-4;20]___UNIQUE_1)
  TransmissionControlUnit/1(Gear[-4;20]) -> DrivetrainControlUnitOutput/1(Gear[-4;20]___UNIQUE_1)
  TransmissionControlUnit/5(ASRRequestSwitch[0;2]) -> DrivetrainControlUnitOutput/5(ASRRequestSwitch[0;2]___UNIQUE_1)
  TransmissionControlUnit/2(LockUpClutchPos[0_1]) -> DrivetrainControlUnitOutput/2(LockUpClutchPos[0_1]___UNIQUE_1)
  TransmissionControlUnit/6(ASRTrq[Nm]) -> DrivetrainControlUnitOutput/6(ASRTrq[Nm]___UNIQUE_1)
  InputFromCTRL/4(InitialGear[-4;20]___UNIQUE_1) -> TransmissionControlUnit/6(InitialGear[-4;20])
  InputFromCTRL/5(MaxGear[-4;20]___UNIQUE_1) -> TransmissionControlUnit/7(MaxGear[-4;20])
  InputFromCTRL/6(MinGear[-4;20]___UNIQUE_1) -> TransmissionControlUnit/8(MinGear[-4;20])
  InputFromCTRL/7(ShiftingProgramSelection[-]___UNIQUE_1) -> TransmissionControlUnit/9(ShiftingProgramSelection[-])
  InputFromCTRL/8(KickdownSwitch[0;1]___UNIQUE_1) -> TransmissionControlUnit/10(KickdownSwitch[0;1])
  Switch/1 -> TransmissionControlUnit/1(AccPedalPos[0_1])
  InputFromCTRL/1(TransmissionLoad[0_1]___UNIQUE_1) -> Switch/1
  InputFromCTRL/2(IntendedEngTrqActive[0;1]___UNIQUE_1) -> Switch/2
  InputFromCTRL/3(AccPedalPos[0_1]___UNIQUE_1) -> Switch/3
  fromEngine/1 -> Terminator/1
  fromDrivetrainPhysics/1 -> InputFromDrivetrainPhysics/1(fromDrivetrainPhysics)
  fromCTRL/1 -> InputFromCTRL/1(fromCTRL)
  InputFromDrivetrainPhysics/3(InSpd[rad/s]___UNIQUE_1) -> TransmissionControlUnit/3(TransmissionInSpd[rad/s])
  InputFromDrivetrainPhysics/1(Type[-]___UNIQUE_1) -> Transmission.Type ~= Manual/1
  InputFromDrivetrainPhysics/5(NumFwdGears[-]___UNIQUE_1) -> TransmissionControlUnit/5(NumFwdGears[-])
  InputFromDrivetrainPhysics/2(EngSpd[rad/s]) -> TransmissionControlUnit/2(EngSpd[rad/s])
  Transmission.Type ~= Manual/1 -> TransmissionControlUnit/Enable
  InputFromDrivetrainPhysics/4(OutSpd[rad/s]___UNIQUE_1) -> TransmissionControlUnit/4(TransmissionOutSpd[rad/s])

== system PassengerCar/Vehicle/Drivetrain/DrivetrainOutputs ==
  DrivetrainPhysics___UNIQUE_1 : Inport  Description=|
      | <name>DrivetrainPhysics</name>
      | <comment></comment>
  DrivetrainControlUnit___UNIQUE_1 : Inport  Description=|  Port=2
      | <name>DrivetrainControlUnit</name>
      | <comment></comment>
  __TDO__Drivetrain : BusCreator  Inputs=2
  Drivetrain___UNIQUE_1 : Outport  Description=|  VectorParamsAs1DForOutWhenUnconnected=off
      | <name>DrivetrainPhysics</name>
      | <comment></comment>
  wires:
  DrivetrainPhysics___UNIQUE_1/1 -> __TDO__Drivetrain/1  "DrivetrainPhysics"
  DrivetrainControlUnit___UNIQUE_1/1 -> __TDO__Drivetrain/2  "DrivetrainControlUnit"
  __TDO__Drivetrain/1 -> Drivetrain___UNIQUE_1/1  "Drivetrain"

== system PassengerCar/Vehicle/Drivetrain/DrivetrainPhysics ==
  fromDrivetrainControlUnit : Inport
  fromCTRL : Inport  Port=2
  fromAuxiliaries : Inport  Port=3
  fromElectricalSystem : Inport  Port=4
  fromEngine : Inport  Port=5
  fromWheelSystem : Inport  Port=6
  DrivetrainPhysicsInputs : Subsystem
  DrivetrainPhysicsOutputs : Subsystem
  DynaComponentInfo : Subsystem  Tag=DynaComponentInfo
      mask init:
      | data= get_param(gcb, 'UserData');
      settings: OpenFcn=DYNA4.ModelHandling.Component.ShowEditComponentInformationDialog(gcb);
      mask Display: disp(['Type = ', data.type, '\nGroup = ', data.group, '\nName = ', data.name ])
  ElasticDrivetrain : DrivetrainModules/ElasticDrivetrain  Tag=vedynaDrivetrainMask  local_comp_inst=1  system_comp_inst=1  DATA_NODE=MDL.Vehicle.Drivetrain.DrivetrainPhysics  sample_time=-1
  Terminator : Terminator
  DrivetrainPhysics : Outport  VectorParamsAs1DForOutWhenUnconnected=off
  wires:
  DrivetrainPhysicsInputs/3(FromEngine) -> ElasticDrivetrain/3
  DrivetrainPhysicsInputs/5(FromWheelSystem) -> ElasticDrivetrain/5
  ElasticDrivetrain/2 -> DrivetrainPhysicsOutputs/2(ShaftStates)
  DrivetrainPhysicsInputs/4(FromCTRL) -> ElasticDrivetrain/4
  DrivetrainPhysicsInputs/1(InitEngSpd[rad/s]) -> ElasticDrivetrain/1
  ElasticDrivetrain/3 -> DrivetrainPhysicsOutputs/3(DrivetrainStates)
  ElasticDrivetrain/1 -> DrivetrainPhysicsOutputs/1(EngStates)
  DrivetrainPhysicsInputs/2(InitialGear[-4;20]) -> ElasticDrivetrain/2
  DrivetrainPhysicsOutputs/1(DrivetrainPhysics) -> DrivetrainPhysics/1
  fromEngine/1 -> DrivetrainPhysicsInputs/1(fromEngine)
  fromWheelSystem/1 -> DrivetrainPhysicsInputs/2(fromWheelSystem)
  fromCTRL/1 -> DrivetrainPhysicsInputs/3(fromCTRL)
  fromDrivetrainControlUnit/1 -> DrivetrainPhysicsInputs/4(fromDrivetrainControlUnit)
  fromAuxiliaries/1 -> DrivetrainPhysicsInputs/5(fromAuxiliaries)
  fromElectricalSystem/1 -> Terminator/1

== system PassengerCar/Vehicle/Drivetrain/DynaComponentInfo ==

== system PassengerCar/Vehicle/ElectricalSystem/DynaComponentInfo ==

== system PassengerCar/Vehicle/ElectricalSystem/ElectricalSystemOutput ==
  LowVoltageBattery___UNIQUE_1 : Inport  Description=|
      | <name>LowVoltageBattery</name>
      | <comment>Voltage level of low voltage battery</comment>
  StarterVoltage[V]___UNIQUE_1 : Inport  Description=|  Port=2  PortDimensions=[1]
      | <name>StarterVoltage[V]</name>
      | <comment>Voltage level of starter</comment>
  GeneratorVoltage[V]___UNIQUE_1 : Inport  Description=|  Port=3  PortDimensions=[1]
      | <name>GeneratorVoltage[V]</name>
      | <comment>Voltage level of generator</comment>
  __TDD__ElectricalSystem.GeneratorVoltage[V] : Demux  Outputs=[1]
  __TDD__ElectricalSystem.StarterVoltage[V] : Demux  Outputs=[1]
  __TDO__ElectricalSystem : BusCreator  Inputs=3
  ElectricalSystem___UNIQUE_1 : Outport  Description=|  VectorParamsAs1DForOutWhenUnconnected=off
      | <name>LowVoltageBattery</name>
      | <comment>Voltage level of low voltage battery</comment>
  wires:
  __TDO__ElectricalSystem/1 -> ElectricalSystem___UNIQUE_1/1  "ElectricalSystem"
  __TDD__ElectricalSystem.GeneratorVoltage[V]/1 -> __TDO__ElectricalSystem/3  "GeneratorVoltage[V]"
  GeneratorVoltage[V]___UNIQUE_1/1 -> __TDD__ElectricalSystem.GeneratorVoltage[V]/1
  __TDD__ElectricalSystem.StarterVoltage[V]/1 -> __TDO__ElectricalSystem/2  "StarterVoltage[V]"
  StarterVoltage[V]___UNIQUE_1/1 -> __TDD__ElectricalSystem.StarterVoltage[V]/1
  LowVoltageBattery___UNIQUE_1/1 -> __TDO__ElectricalSystem/1  "LowVoltageBattery"

== system PassengerCar/Vehicle/ElectricalSystem/LowVoltageBatteryOutput ==
  LowVoltageBatteryVoltage[V]___UNIQUE_1 : Inport  Description=|  PortDimensions=[1]
      | <name>LowVoltageBatteryVoltage[V]</name>
      | <comment>RMS voltage at inverter output</comment>
  LowVoltageBatterySOC[0_1]___UNIQUE_1 : Inport  Description=|  Port=2  PortDimensions=[1]
      | <name>LowVoltageBatterySOC[0_1]</name>
      | <comment>Current at inverter input</comment>
  __TDD__LowVoltageBattery.LowVoltageBatterySOC[0_1] : Demux  Outputs=[1]
  __TDD__LowVoltageBattery.LowVoltageBatteryVoltage[V] : Demux  Outputs=[1]
  __TDO__LowVoltageBattery : BusCreator  Inputs=2
  LowVoltageBattery___UNIQUE_1 : Outport  Description=|  PortDimensions=[2]  VectorParamsAs1DForOutWhenUnconnected=off
      | <name>LowVoltageBatteryVoltage[V]</name>
      | <comment>RMS voltage at inverter output</comment>
  wires:
  __TDO__LowVoltageBattery/1 -> LowVoltageBattery___UNIQUE_1/1  "LowVoltageBattery"
  __TDD__LowVoltageBattery.LowVoltageBatterySOC[0_1]/1 -> __TDO__LowVoltageBattery/2  "LowVoltageBatterySOC[0_1]"
  LowVoltageBatterySOC[0_1]___UNIQUE_1/1 -> __TDD__LowVoltageBattery.LowVoltageBatterySOC[0_1]/1
  __TDD__LowVoltageBattery.LowVoltageBatteryVoltage[V]/1 -> __TDO__LowVoltageBattery/1  "LowVoltageBatteryVoltage[V]"
  LowVoltageBatteryVoltage[V]___UNIQUE_1/1 -> __TDD__LowVoltageBattery.LowVoltageBatteryVoltage[V]/1

== system PassengerCar/Vehicle/Engine/DynaComponentInfo ==
